simulink model "Simulink1"  (R2022a)
settings: Solver=VariableStepAuto  StartTime=0.0  StopTime=10.0  RelTol=1e-3
settings Model: Creator=a2270340  LastModifiedBy=a2270340

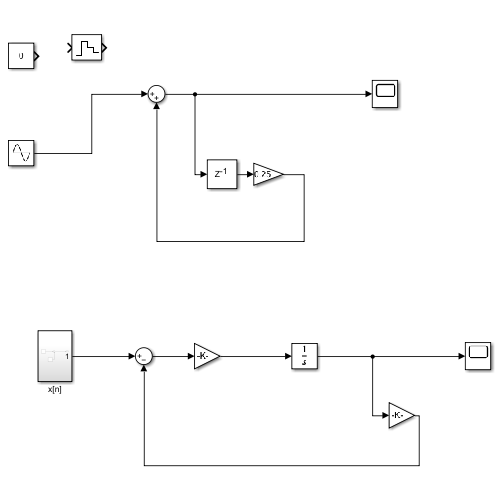
[thumbnail: Simulink's stored preview of the top-level diagram]
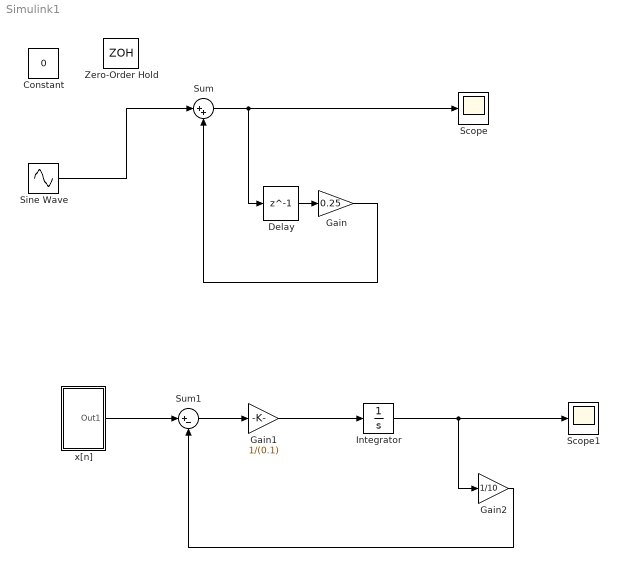
== system Simulink1 ==
  Constant : Constant  Value=0
  Delay : Delay  DelayLength=1  InitialCondition=-8
  Gain : Gain  Gain=0.25
  Gain1 : Gain  Gain=1/(0.1)
  Gain2 : Gain  Gain=1/10
  Integrator : Integrator
  Scope : Scope
  Scope1 : Scope
  Sine Wave : Sin  Frequency=9*pi/10  SampleTime=0
  Sum : Sum  Inputs=|++
  Sum1 : Sum  Inputs=|+-
  Zero-Order Hold : ZeroOrderHold
  x[n] : Subsystem
  wires:
  Sum/1 -> Delay/1, Scope/1
  Delay/1 -> Gain/1
  Gain/1 -> Sum/2
  Sine Wave/1 -> Sum/1
  Gain1/1 -> Integrator/1
  Sum1/1 -> Gain1/1
  x[n]/1(Out1) -> Sum1/1
  Gain2/1 -> Sum1/2
  Integrator/1 -> Scope1/1, Gain2/1

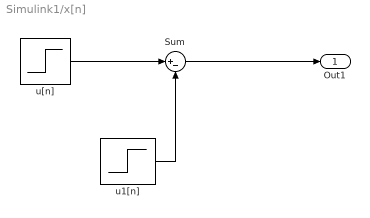
== system Simulink1/x[n] ==
  Sum : Sum  Inputs=|+-
  u1[n] : Step  Time=5  SampleTime=0
  u[n] : Step  SampleTime=0
  Out1 : Outport
  wires:
  u[n]/1 -> Sum/1
  u1[n]/1 -> Sum/2
  Sum/1 -> Out1/1
